simulink model "get_data_from_xplane_9"  (R2016a)
settings: Solver=VariableStepAuto  StartTime=0.0  StopTime=inf  RelTol=1e-3
libraries: dspindex x8, dspnetwork x1
settings Model: Creator=iwin  LastModifiedBy=iwin

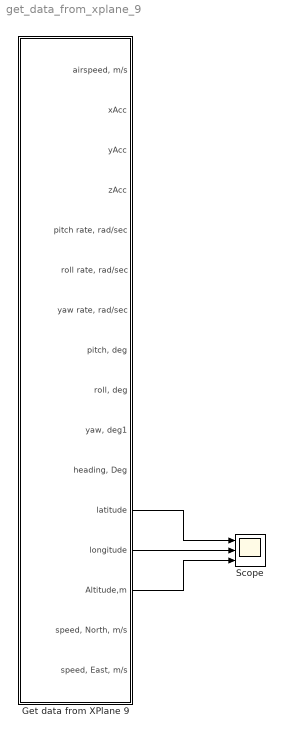
== system get_data_from_xplane_9 ==
  Get data from XPlane 9 : Subsystem  Description=|  TreatAsAtomicUnit=on  mask(Get Data from Xplane10){remoteURL='192.168.137.129', localPort=49005, sampletime=0.02}
      | Done by: Mohamed Abdelkader
      | Contact for updates: mohamedashraf123@gmail.com
      mask prompts: remoteURL "Remote IP address ('0.0.0.0' to accept all):(default='127.0.0.1')"; localPort "Local IP port: that Xplane10 sends to (default=49005)"; sampletime "Sampling time (seconds), how frequenlty to capture data from Xplane. Don't set to low as it might not be able to capture the smaples from Xplane. Default is 0.02 assuming the UDP rate in Xplane is set to 50 sample per second"
      mask help:
      | Get Data from X-Plane10
      | * make sure you configure the right port
      | and the right IP address
      mask TypeOptions remoteURL: UDP Receive1/remoteURL
      mask TypeOptions localPort: UDP Receive1/localPort
      mask TypeOptions sampletime: UDP Receive1/sampletime
  Scope : Scope  NumInputPorts=3
  wires:
  Get data from XPlane 9/13(longitude) -> Scope/2
  Get data from XPlane 9/12(latitude) -> Scope/1
  Get data from XPlane 9/14(Altitude,m) -> Scope/3

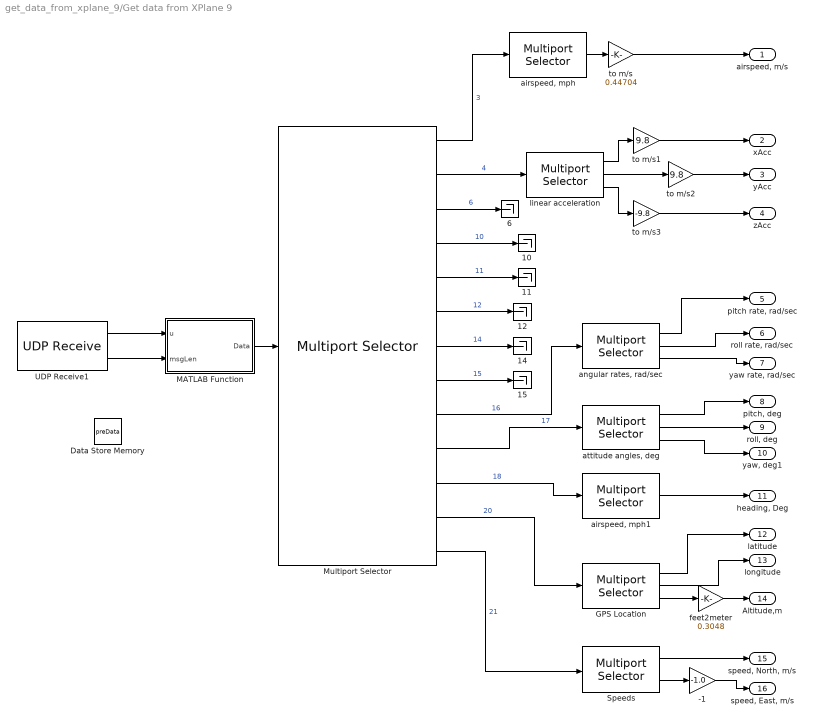
== system get_data_from_xplane_9/Get data from XPlane 9 ==
  -1 : Gain  Gain=-1.0
  {6,10..12,14..15} (6 alike) : Terminator
  Data Store Memory : DataStoreMemory  DataStoreName=preData  InitialValue=zeros(140, 8)  ShowAdditionalParam=off  OutDataTypeStr=single
  GPS Location : dspindex/Multiport Selector  rowsOrCols=Columns  idxCellArray={1,2,4}  idxErrMode=Clip Index
  MATLAB Function : MATLAB Function  TreatAsAtomicUnit=on
  Multiport Selector : dspindex/Multiport Selector  rowsOrCols=Rows  idxCellArray={3,4,6,10,11,12,14,15,16,17,18,20,21}  idxErrMode=Clip Index
  Speeds : dspindex/Multiport Selector  rowsOrCols=Columns  idxCellArray={4,6}  idxErrMode=Clip Index
  UDP Receive1 : dspnetwork/UDP Receive  localURL='0.0.0.0'  localPort=localPort  remoteURL=remoteURL  remotePort=-1  recvBufferSize=8192  dims=365*20  signalDatatype=uint8  isVarSize=off  showBlockingTime=off  blockingTime=0  sampletime=sampletime
  "airspeed, mph" : dspindex/Multiport Selector  rowsOrCols=Columns  idxCellArray={6}  idxErrMode=Clip Index
  "airspeed, mph1" : dspindex/Multiport Selector  rowsOrCols=Columns  idxCellArray={3}  idxErrMode=Clip Index
  "angular rates, rad/sec" : dspindex/Multiport Selector  rowsOrCols=Columns  idxCellArray={1,2,3}  idxErrMode=Clip Index
  "attitude angles, deg" : dspindex/Multiport Selector  rowsOrCols=Columns  idxCellArray={1,2,3}  idxErrMode=Clip Index
  feet2meter : Gain  Gain=0.3048
  linear acceleration : dspindex/Multiport Selector  rowsOrCols=Columns  idxCellArray={6,7,5}  idxErrMode=Clip Index
  to m/s : Gain  Gain=0.44704
  to m/s1 : Gain  Gain=9.8
  to m/s2 : Gain  Gain=9.8
  to m/s3 : Gain  Gain=-9.8
  "airspeed, m/s" : Outport
  xAcc : Outport  Port=2
  yAcc : Outport  Port=3
  zAcc : Outport  Port=4
  "pitch rate, rad/sec" : Outport  Port=5
  "roll rate, rad/sec" : Outport  Port=6
  "yaw rate, rad/sec" : Outport  Port=7
  "pitch, deg " : Outport  Port=8
  "roll, deg" : Outport  Port=9
  "yaw, deg1" : Outport  Port=10
  "heading, Deg" : Outport  Port=11
  latitude : Outport  Port=12
  longitude : Outport  Port=13
  Altitude,m : Outport  Port=14
  "speed, North, m/s" : Outport  Port=15
  "speed, East, m/s" : Outport  Port=16
  wires:
  UDP Receive1/2 -> MATLAB Function/2(msgLen)
  UDP Receive1/1 -> MATLAB Function/1(u)
  -1/1 -> "speed, East, m/s"/1
  feet2meter/1 -> Altitude,m/1
  to m/s3/1 -> zAcc/1
  "airspeed, mph1"/1 -> "heading, Deg"/1
  Multiport Selector/11 -> "airspeed, mph1"/1  "18"
  Multiport Selector/10 -> "attitude angles, deg"/1  "17"
  Speeds/2 -> -1/1
  "angular rates, rad/sec"/2 -> "roll rate, rad/sec"/1
  linear acceleration/3 -> to m/s3/1
  "angular rates, rad/sec"/1 -> "pitch rate, rad/sec"/1
  Speeds/1 -> "speed, North, m/s"/1
  GPS Location/1 -> latitude/1
  linear acceleration/1 -> to m/s1/1
  Multiport Selector/12 -> GPS Location/1  "20"
  "airspeed, mph"/1 -> to m/s/1
  Multiport Selector/13 -> Speeds/1  "21"
  Multiport Selector/6 -> 12/1  "12"
  to m/s/1 -> "airspeed, m/s"/1
  Multiport Selector/4 -> 10/1  "10"
  GPS Location/3 -> feet2meter/1
  "attitude angles, deg"/2 -> "roll, deg"/1
  "attitude angles, deg"/1 -> "pitch, deg "/1
  to m/s1/1 -> xAcc/1
  to m/s2/1 -> yAcc/1
  linear acceleration/2 -> to m/s2/1
  GPS Location/2 -> longitude/1
  Multiport Selector/8 -> 15/1  "15"
  Multiport Selector/1 -> "airspeed, mph"/1  "3"
  MATLAB Function/1(Data) -> Multiport Selector/1
  "angular rates, rad/sec"/3 -> "yaw rate, rad/sec"/1
  Multiport Selector/7 -> 14/1  "14"
  "attitude angles, deg"/3 -> "yaw, deg1"/1
  Multiport Selector/9 -> "angular rates, rad/sec"/1  "16"
  Multiport Selector/3 -> 6/1  "6"
  Multiport Selector/2 -> linear acceleration/1  "4"
  Multiport Selector/5 -> 11/1  "11"

== matlab function get_data_from_xplane_9/Get data from XPlane 9/MATLAB Function ==
  data: u input uint8; Data output single size=[140 8]; msgLen input; preData data_store_memory
% 
% Handle the data received from x-plane 9
% 
% Author: Gui Zhou
% Date: 2017-02-14
%

function Data  = fcn(u,msgLen)
    %#codegen
    global preData; 
    %coder.extrinsic('clear')
    dataLen=msgLen-5;
    Npackets=dataLen/36; 
    % initialize data matrix
    % rows: packets of data; columns: data values, first column is the data
    % index  



    maxNPackets=140;
    Nvalues=8;% number of values in each packet
    Data=single(zeros(maxNPackets,Nvalues));

    if dataLen ~= 0 

        Bytecounter=6; % start after the 5th byte 
        for j=1:Npackets
                        indx=typecast(u(Bytecounter:Bytecounter+3),'uint32');% packet index
                        %Data(indx,1)=single(indx); % packet index
                        Bytecounter=Bytecounter+4; % go to the next 4 bytes
                        Data(indx,1)=typecast(u(Bytecounter:Bytecounter+3),'single'); % 1st value
                        Bytecounter=Bytecounter+4; % go to the next 4 bytes
                        Data(indx,2)=typecast(u(Bytecounter:Bytecounter+3),'single'); % 2nd value
                        Bytecounter=Bytecounter+4; % go to the next 4 bytes
                        Data(indx,3)=typecast(u(Bytecounter:Bytecounter+3),'single'); % 3rd value
                        Bytecounter=Bytecounter+4; % go to the next 4 bytes
                        Data(indx,4)=typecast(u(Bytecounter:Bytecounter+3),'single'); % 4th value
                        Bytecounter=Bytecounter+4; % go to the next 4 bytes
                        Data(indx,5)=typecast(u(Bytecounter:Bytecounter+3),'single'); % 5th value
                        Bytecounter=Bytecounter+4; % go to the next 4 bytes
                        Data(indx,6)=typecast(u(Bytecounter:Bytecounter+3),'single'); % 6th value
                        Bytecounter=Bytecounter+4; % go to the next 4 bytes
                        Data(indx,7)=typecast(u(Bytecounter:Bytecounter+3),'single'); % 7th value
                        Bytecounter=Bytecounter+4; % go to the next 4 bytes
                        Data(indx,8)=typecast(u(Bytecounter:Bytecounter+3),'single'); % 8th value
                        Bytecounter=Bytecounter+4;% go to the next packet index 
        end  
        
        preData = Data;

    else 

        Data = preData;

            
    end
end



%clear Data
